simulink model "mass_spring_damper_simulink_simscape_project_solution"  (R2022a)
settings: Solver=VariableStepAuto  StartTime=0.0  StopTime=30  FixedStep=0.01  RelTol=1e-3  AbsTol=1e-3
undefined symbols (not defined in the file): b1, b2, k1, k2, m1, m2
libraries: fl_lib x14, nesl_utility x5
settings Model: Creator=Dr. Ryan Aly  LastModifiedBy=Dr. Ryan Aly
settings SolverCC: AutoScaleAbsTol=off  AlgebraicLoopSolver=TrustRegion  MaxZcPerStep=1
settings DataIOCC: ReturnWorkspaceOutputs=off  Refine=10
settings DebuggingCC: UnconnectedInputMsg=warning  UnconnectedOutputMsg=warning  UnconnectedLineMsg=warning  SymbolicDimsDataTypeCodeGenerationDiagnostic=none  SFMachineParentedDataDiag=warning
settings SFSimCC: CustomCodeUndefinedFunction=UseInterfaceOnly
settings RTWCC: DLArmComputeVersion=19.05
settings SimscapeCC: SimscapeLogType=all  SimscapeLogSimulationStatistics=on  SimscapeLogDataHistory=10000

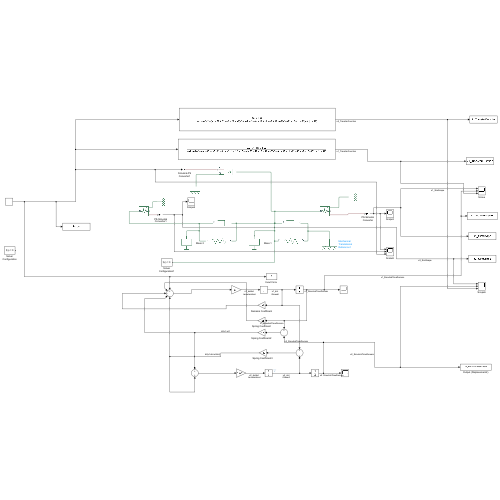
[thumbnail: Simulink's stored preview of the top-level diagram]
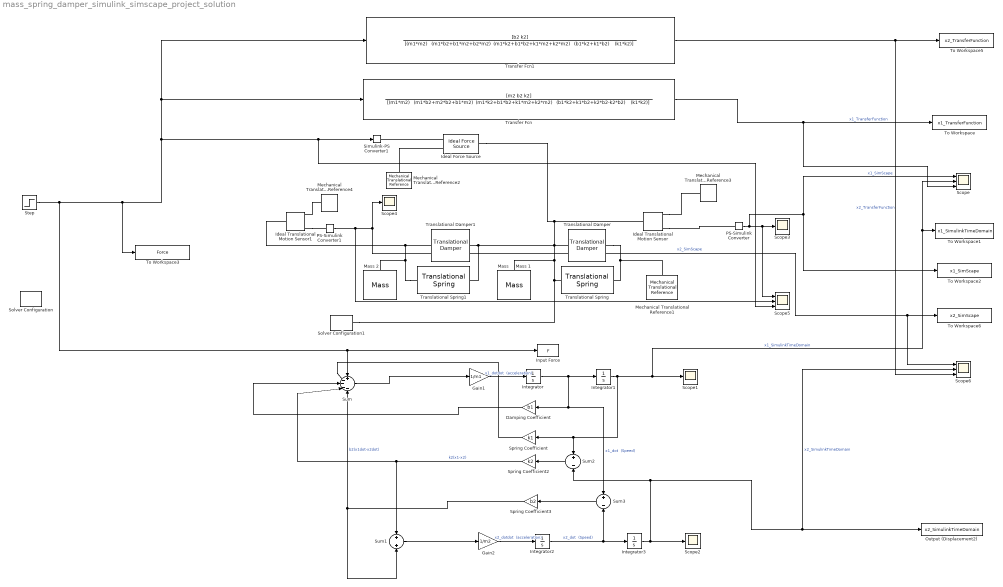
== system mass_spring_damper_simulink_simscape_project_solution ==
  Damping Coefficient : Gain  Gain=b1
  Gain1 : Gain  Gain=1/m1
  Gain2 : Gain  Gain=1/m2
  Ideal Force Source : fl_lib/Mechanical/Mechanical Sources/Ideal Force Source
      settings: SourceProductBaseCode=PW,SS,VE
  Ideal Translational Motion Sensor : fl_lib/Mechanical/Mechanical Sensors/Ideal Translational Motion Sensor  offset=0 m
      settings: SourceProductBaseCode=PW,SS,VE
  Ideal Translational Motion Sensor1 : fl_lib/Mechanical/Mechanical Sensors/Ideal Translational Motion Sensor  offset=0 m
      settings: SourceProductBaseCode=PW,SS,VE
  Input Force : ToWorkspace  VariableName=F  SaveFormat=Timeseries  SampleTime=-1
  Integrator{,1..3} (4 alike) : Integrator
  Mass : fl_lib/Mechanical/Translational Elements/Mass  mass=1 kg  num_ports=foundation.enum.numPorts2.one  v_specify=off  v_priority=High  v=0 m/s  v_nominal_specify=off  v_nominal_unit=m/s  v_nominal_value=1  f_specify=off  f_priority=None  f=0 N  f_nominal_specify=off  f_nominal_unit=N  f_nominal_value=1
      settings: SourceProductBaseCode=PW,SS,VE
  Mass 1 : fl_lib/Mechanical/Translational Elements/Mass  mass=m1 kg  num_ports=foundation.enum.numPorts2.one  v_specify=off  v_priority=High  v=0 m/s  v_nominal_specify=off  v_nominal_unit=m/s  v_nominal_value=1  f_specify=off  f_priority=None  f=0 N  f_nominal_specify=off  f_nominal_unit=N  f_nominal_value=1
      settings: SourceProductBaseCode=PW,SS,VE
  Mass 2 : fl_lib/Mechanical/Translational Elements/Mass  mass=m2 kg  num_ports=foundation.enum.numPorts2.one  v_specify=off  v_priority=High  v=0 m/s  v_nominal_specify=off  v_nominal_unit=m/s  v_nominal_value=1  f_specify=off  f_priority=None  f=0 N  f_nominal_specify=off  f_nominal_unit=N  f_nominal_value=1
      settings: SourceProductBaseCode=PW,SS,VE
  Mechanical Translational Reference{1..4} (4 alike) : fl_lib/Mechanical/Translational Elements/Mechanical Translational Reference
      settings: SourceProductBaseCode=PW,SS,VE
  Output (Displacement2) : ToWorkspace  VariableName=x2_SimulinkTimeDomain  SaveFormat=Timeseries  SampleTime=-1
  PS-Simulink Converter : nesl_utility/PS-Simulink Converter  PhysicalDomain=network_engine_domain  SubClassName=ps_output  LeftPortType=input  RightPortType=output  PseudoPeriodic=off  Frequencies=[]  VectorFormat=inherit  Unit=inherit  AffineConversion=off
      settings: SourceProductBaseCode=SS,PW,VE
  PS-Simulink Converter1 : nesl_utility/PS-Simulink Converter  PhysicalDomain=network_engine_domain  SubClassName=ps_output  LeftPortType=input  RightPortType=output  PseudoPeriodic=off  Frequencies=[]  VectorFormat=inherit  Unit=inherit  AffineConversion=off
      settings: SourceProductBaseCode=SS,PW,VE
  Scope : Scope  NumInputPorts=3
  Scope{1..4} (4 alike) : Scope
  Scope5 : Scope  NumInputPorts=3
  Scope6 : Scope  NumInputPorts=3
  Simulink-PS Converter1 : nesl_utility/Simulink-PS Converter  PhysicalDomain=network_engine_domain  SubClassName=ps_input  LeftPortType=input  RightPortType=output  PseudoPeriodic=off  Frequencies=[]  NoiseDistribution=none  NoiseParameters=[]  Unit=1  AffineConversion=off  FilteringAndDerivatives=provide  SimscapeFilterOrder=1  InputFilterTimeConstant=0.001  UdotUserProvided=0
      settings: SourceProductBaseCode=SS,PW,VE
  Solver Configuration : nesl_utility/Solver Configuration  PhysicalDomain=network_engine_domain  SubClassName=solver  LeftPortType=input  RightPortType=generic  Tones=[]  Harmonics=[]  SimulateNoise=off  Profile=off  UseLocalSampling=off  EnableSwitchedLinearOptims=on  FrequencyDomain=off  UseCCode=off  RelTol=0.001  AbsTol=1e-06  MinStep=1e-09  ToWorkspace=off  RevertToSquareIcSolve=off  NumHomotopyIterations=100  PhasorMode=off  PhasorModeNumHarmonics=1  IndexReductionMethod=DerivativeReplacement  DoDC=off  ResidualTolerance=1e-09  UseLocalSolver=off  LocalSolverChoice=NE_BACKWARD_EULER_ADVANCER  LocalSolverSampleTime=0.001  DoFixedCost=off  MaxNonlinIter=3  MaxModeIter=2  ComputeImpulses=off  ImpulseIterations=2  LinearAlgebra=auto  LinearAlgebraNumThread=0  EquationFormulation=NE_TIME_EF  DelaysMemoryBudget=1024  AutomaticFiltering=on  FilteringTimeConstant=0.001  PartitionStorageMethod=AS_NEEDED  PartitionMemoryBudget=1024  PartitionMethod=ROBUST
      settings: SourceProductBaseCode=SS,PW,VE
  Solver Configuration1 : nesl_utility/Solver Configuration  PhysicalDomain=network_engine_domain  SubClassName=solver  LeftPortType=input  RightPortType=generic  Tones=[]  Harmonics=[]  SimulateNoise=off  Profile=off  UseLocalSampling=off  EnableSwitchedLinearOptims=on  FrequencyDomain=off  UseCCode=off  RelTol=0.001  AbsTol=1e-06  MinStep=1e-09  ToWorkspace=off  RevertToSquareIcSolve=off  NumHomotopyIterations=100  PhasorMode=off  PhasorModeNumHarmonics=1  IndexReductionMethod=DerivativeReplacement  DoDC=off  ResidualTolerance=1e-09  UseLocalSolver=off  LocalSolverChoice=NE_BACKWARD_EULER_ADVANCER  LocalSolverSampleTime=0.001  DoFixedCost=off  MaxNonlinIter=3  MaxModeIter=2  ComputeImpulses=off  ImpulseIterations=2  LinearAlgebra=auto  LinearAlgebraNumThread=0  EquationFormulation=NE_TIME_EF  DelaysMemoryBudget=1024  AutomaticFiltering=on  FilteringTimeConstant=0.001  PartitionStorageMethod=AS_NEEDED  PartitionMemoryBudget=1024  PartitionMethod=ROBUST
      settings: SourceProductBaseCode=SS,PW,VE
  Spring Coefficient : Gain  Gain=k1
  Spring Coefficient2 : Gain  Gain=k2
  Spring Coefficient3 : Gain  Gain=b2
  Step : Step  SampleTime=0
  Sum : Sum  Inputs=+----
  Sum1 : Sum
  Sum2 : Sum  Inputs=+-
  Sum3 : Sum  Inputs=+-
  To Workspace : ToWorkspace  VariableName=x1_TransferFunction  SaveFormat=Timeseries  SampleTime=-1
  To Workspace1 : ToWorkspace  VariableName=x1_SimulinkTimeDomain  SaveFormat=Timeseries  SampleTime=-1
  To Workspace2 : ToWorkspace  VariableName=x1_SimScape  SaveFormat=Timeseries  SampleTime=-1
  To Workspace3 : ToWorkspace  VariableName=Force  SaveFormat=Timeseries  SampleTime=-1
  To Workspace5 : ToWorkspace  VariableName=x2_TransferFunction  SaveFormat=Timeseries  SampleTime=-1
  To Workspace6 : ToWorkspace  VariableName=x2_SimScape  SaveFormat=Timeseries  SampleTime=-1
  Transfer Fcn : TransferFcn  Numerator=[m2 b2 k2]  Denominator="[(m1*m2)   (m1*b2+m2*b2+b1*m2)  (m1*k2+b1*b2+k1*m2+k2*m2)   (b1*k2+k1*b2+k2*b2-k2*b2)    (k1*k2)]"
  Transfer Fcn1 : TransferFcn  Numerator=[b2 k2]  Denominator="[(m1*m2)   (m1*b2+b1*m2+b2*m2)  (m1*k2+b1*b2+k1*m2+k2*m2)   (b1*k2+k1*b2)    (k1*k2)]"
  Translational Damper : fl_lib/Mechanical/Translational Elements/Translational Damper  D=b1 N*s/m  v_specify=off  v_priority=None  v=0 m/s  v_nominal_specify=off  v_nominal_unit=m/s  v_nominal_value=1  f_specify=off  f_priority=None  f=0 N  f_nominal_specify=off  f_nominal_unit=N  f_nominal_value=1
      settings: SourceProductBaseCode=PW,SS,VE
  Translational Damper1 : fl_lib/Mechanical/Translational Elements/Translational Damper  D=b2 N*s/m  v_specify=off  v_priority=None  v=0 m/s  v_nominal_specify=off  v_nominal_unit=m/s  v_nominal_value=1  f_specify=off  f_priority=None  f=0 N  f_nominal_specify=off  f_nominal_unit=N  f_nominal_value=1
      settings: SourceProductBaseCode=PW,SS,VE
  Translational Spring : fl_lib/Mechanical/Translational Elements/Translational Spring  spr_rate=k1 N/m  v_specify=off  v_priority=None  v=0 m/s  v_nominal_specify=off  v_nominal_unit=m/s  v_nominal_value=1  f_specify=off  f_priority=None  f=0 N  f_nominal_specify=off  f_nominal_unit=N  f_nominal_value=1  x_specify=off  x_priority=High  x=0 m  x_nominal_specify=off  x_nominal_unit=m  x_nominal_value=1
      settings: SourceProductBaseCode=PW,SS,VE
  Translational Spring1 : fl_lib/Mechanical/Translational Elements/Translational Spring  spr_rate=k2 N/m  v_specify=off  v_priority=None  v=0 m/s  v_nominal_specify=off  v_nominal_unit=m/s  v_nominal_value=1  f_specify=off  f_priority=None  f=0 N  f_nominal_specify=off  f_nominal_unit=N  f_nominal_value=1  x_specify=off  x_priority=High  x=0 m  x_nominal_specify=off  x_nominal_unit=m  x_nominal_value=1
      settings: SourceProductBaseCode=PW,SS,VE
  wires:
  PS-Simulink Converter/1 -> Scope5/1, Scope3/1, Scope/1, To Workspace2/1  "x1_SimScape"
  Integrator1/1 -> Sum2/1, Spring Coefficient/1, Scope/2, To Workspace1/1, Scope1/1  "x1_SimulinkTimeDomain"
  Transfer Fcn/1 -> To Workspace/1, Scope/3  "x1_TransferFunction"
  Sum3/1 -> Spring Coefficient3/1
  Sum/1 -> Gain1/1
  Spring Coefficient2/1 -> Sum/4, Sum1/1  "k2(x1-x2)"
  Spring Coefficient3/1 -> Sum1/2, Sum/5  "b2(x1dot-x2dot)"
  Integrator3/1 -> Scope2/1, Sum2/2, Output (Displacement2)/1, Scope6/2  "x2_SimulinkTimeDomain"
  Integrator/1 -> Sum3/1, Damping Coefficient/1, Integrator1/1  "x1_dot  (Speed)"
  Spring Coefficient/1 -> Sum/2
  Damping Coefficient/1 -> Sum/3
  Sum1/1 -> Gain2/1
  Gain2/1 -> Integrator2/1  "x2_dotdot  (acceleration)"
  Sum2/1 -> Spring Coefficient2/1
  Integrator2/1 -> Sum3/2, Integrator3/1  "x2_dot  (Speed)"
  Gain1/1 -> Integrator/1  "x1_dotdot  (acceleration)"
  PS-Simulink Converter1/1 -> Scope5/2, Scope6/1, To Workspace6/1, Scope4/1  "x2_SimScape"
  Step/1 -> Input Force/1, Sum/1, To Workspace3/1, Scope5/3, Simulink-PS Converter1/1, Transfer Fcn1/1, Transfer Fcn/1
  Transfer Fcn1/1 -> To Workspace5/1, Scope6/3  "x2_TransferFunction"
  connections:
  Translational Spring1/LConn1 -- Mass 2/LConn1 -- Translational Damper1/LConn1 -- Ideal Translational Motion Sensor1/LConn1
  Translational Spring/LConn1 -- Solver Configuration1/RConn1 -- Mass/LConn1 -- Ideal Translational Motion Sensor/LConn1 -- Ideal Force Source/LConn1 -- Translational Damper/LConn1 -- Translational Damper1/RConn1 -- Translational Spring1/RConn1
  Translational Spring/RConn1 -- Translational Damper/RConn1 -- Mechanical Translational Reference1/LConn1
  Ideal Translational Motion Sensor1/RConn1 -- Mechanical Translational Reference4/LConn1
  Ideal Force Source/RConn1 -- Simulink-PS Converter1/RConn1
  Ideal Translational Motion Sensor/RConn1 -- Mechanical Translational Reference3/LConn1
  Ideal Translational Motion Sensor1/RConn3 -- PS-Simulink Converter1/LConn1
  Mechanical Translational Reference2/LConn1 -- Ideal Force Source/RConn2
  Ideal Translational Motion Sensor/RConn3 -- PS-Simulink Converter/LConn1
